simulink model "Bordesv2"  (R2022a)
settings: Solver=VariableStepAuto  StartTime=0.0  StopTime=inf  RelTol=1e-3
undefined symbols (not defined in the file or in its folder): none, videoinput
libraries: imaqlib x1, visionconversions x1
settings Model: Creator=jonathan  LastModifiedBy=jonathan

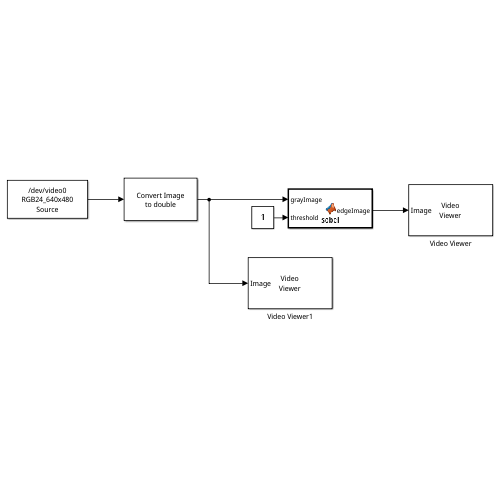
[thumbnail: Simulink's stored preview of the top-level diagram]
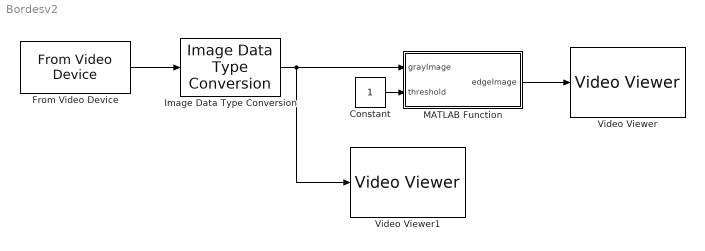
== system Bordesv2 ==
  Constant : Constant
  From Video Device : imaqlib/From Video Device  DeviceMenu=linuxvideo 1 (/dev/video0)  Device=linuxvideo 1 (/dev/video0)  ObjConstructor=videoinput('linuxvideo', 1)  VideoFormatMenu=RGB24_640x480  VideoFormat=RGB24_640x480  VideoSource=Source  ROIPosition=[0 0 480 640]  EnableHWTrigger=off  TriggerConfiguration=none/none  SampleTime=1/30  OutputPortsMode=One multidimensional signal  DataType=single  CanDoHWTrigger=no  ReturnedColorSpace=grayscale  BlockHandle=4.0002  ROIWidth=640  ROIHeight=480  ROIColumn=0  ROIRow=0  EngXMLPath=/usr/local/MATLAB/R2022a/toolbox/imaq/imaq/private  DevXMLPath=/home/jonathan/Documents/MATLAB/SupportPackages/R2022a/toolbox/imaq/supportpackages/genericvideo/adaptor/glnxa64  EngLibPath=/usr/local/MATLAB/R2022a/toolbox/imaq/imaqblks/imaqmex/glnxa64  ColorSpace=grayscale  BayerSensorAlignment=grbg  ImaqMode=off
  Image Data Type Conversion : visionconversions/Image Data Type Conversion  outDT=double  isSigned=on  wordLen=16  numFracBits=0
      settings: SourceProductBaseCode=VP
  MATLAB Function : MATLAB Function  TreatAsAtomicUnit=on
  Video Viewer : VideoViewer  FigPos=[-76 929 1332 608]
  Video Viewer1 : VideoViewer  FigPos=[965 624 406 300]
  wires:
  From Video Device/1 -> Image Data Type Conversion/1
  Image Data Type Conversion/1 -> MATLAB Function/1(grayImage), Video Viewer1/1
  MATLAB Function/1(edgeImage) -> Video Viewer/1
  Constant/1 -> MATLAB Function/2(threshold)

== matlab function Bordesv2/MATLAB Function ==
  data: grayImage input; edgeImage output; threshold input
function edgeImage  = sobel(grayImage,threshold)   %#codegen

% Define Kernel for Sobel edge detection
k = single([1 2 1; 0 0 0; -1 -2 -1]);

% Detect Edge
H = conv2(single(grayImage),k, 'same');
V = conv2(single(grayImage),k','same');
E = sqrt(H.*H + V.*V);
edgeImage = uint8((E > threshold) * 255);

end
